simulink subsystem "rss_ActElecAgElecSpdCmptSens"  (R2023a)
settings: Solver=VariableStepAuto  StartTime=0.0  StopTime=10.0  RelTol=1e-3
libraries: lib_finite_difference_derivative x1
settings Model: DefaultTestHarness=rss_ActualAngleAndSpeedComputation_SensorBased_thu  Creator=CAV2OFO  LastModifiedBy=xiaoqiang.yuan
settings OptimizationCC: ReuseModelBlockBuffer=off

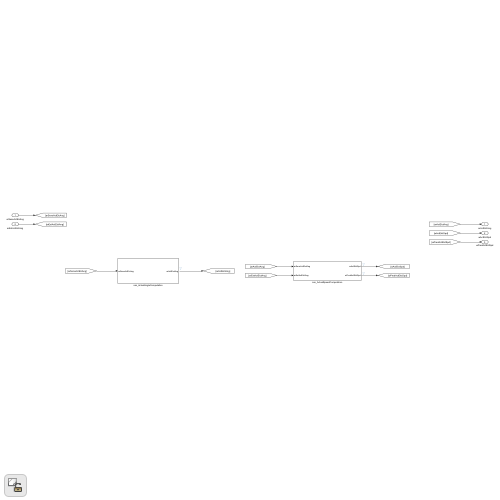
[thumbnail: Simulink's stored preview of the top-level diagram]
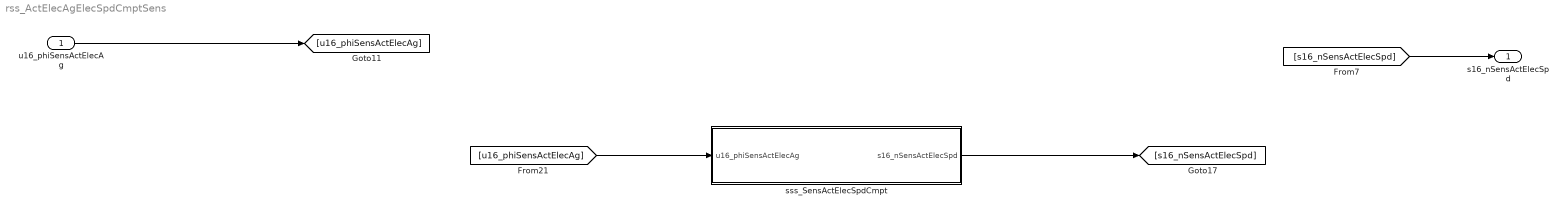
== system rss_ActElecAgElecSpdCmptSens ==
  u16_phiSensActElecAg : Inport  OutDataTypeStr=dt_RadAng_u16r15b0
  sss_SensActElecSpdCmpt : Subsystem
  s16_nSensActElecSpd : Outport  OutDataTypeStr=dt_Standardize_s16p15b0
  wires:
  [u16_phiSensActElecAg] -> sss_SensActElecSpdCmpt/1(u16_phiSensActElecAg)
  sss_SensActElecSpdCmpt/1(s16_nSensActElecSpd) -> [s16_nSensActElecSpd]
  u16_phiSensActElecAg/1 -> [u16_phiSensActElecAg]
  [s16_nSensActElecSpd] -> s16_nSensActElecSpd/1

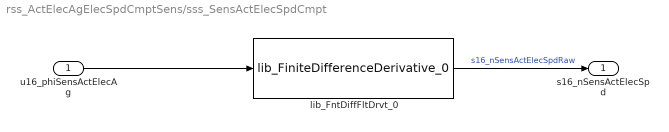
== system rss_ActElecAgElecSpdCmptSens/sss_SensActElecSpdCmpt ==
  u16_phiSensActElecAg : Inport
  lib_FntDiffFltDrvt_0 : lib_finite_difference_derivative/lib_FiniteDifferenceDerivative_0  lb_parSampTime=Cdbl_tiMedTaskSmpTi  lb_parMaxInpVar=Cdbl_phiMaxMedTaskElecAgVrnt  lb_parOutpPhyPek=Cdbl_nElecAgSpdPeakVal  lb_parAngInpMode=on  lb_parOutpDataType=dt_Standardize_s16p15b0
      link override vss_AngleModeSelection: VariantControlMode=label  LabelModeActiveChoice=lb_parAngInpModeLbl
  s16_nSensActElecSpd : Outport
  wires:
  lib_FntDiffFltDrvt_0/1 -> s16_nSensActElecSpd/1  "s16_nSensActElecSpdRaw"
  u16_phiSensActElecAg/1 -> lib_FntDiffFltDrvt_0/1
